simulink model "project_review_simulink"  (R2025b)
settings: Solver=ode4  StartTime=0.0  StopTime=5000  FixedStep=0.01  RelTol=1e-3
values from neighbouring files (symbols this model uses):
  a = 6900    [project_review.m]
  A_BN0 = eye(3)    [project_review.m]
  e = 0.01    [project_review.m]
  e_sun = deg2rad(23.45)    [project_review.m]
  inc = deg2rad(10)    [project_review.m]
  n = sqrt(mu_E / (a^3))    [project_review.m]
  n_sun = 2*pi / T_sun    (= 1.99102127766e-07)    [project_review.m]
  R_sun = 1.496e8    (= 149600000)    [project_review.m]
  sens_gyro_D_bias_inst = 0.3 / 3600    (= 8.33333333333e-05)    [project_review.m]
  sens_gyro_D_RW = sens_gyro_RRW / sqrt(3600)    [project_review.m]
  sens_gyro_D_wn = sens_gyro_D_ARW / sqrt(3600)    [project_review.m]
  sens_gyro_O = [1,      sens_gyro_eps_xy, sens_gyro_eps_xz ... (first row only)    [project_review.m]
  sens_gyro_run_run_bias = 4 / 3600    (= 0.00111111111111)    [project_review.m]
  sens_gyro_SFE = 500 * 1e-6    (= 0.0005)    [project_review.m]
  sens_gyro_SFN = 15 * 1e-6    (= 1.5e-05)    [project_review.m]
  sens_gyro_static_temp_bias = 9 / 3600    (= 0.0025)    [project_review.m]
  sens_gyro_theta_eps = [0,            -sens_gyro_theta_eps_z,  sens_gyro_theta_eps_y ... (first row only)    [project_review.m]
  sens_gyro_Ts = 1 / sens_gyro_update_rate    (= 0.01)    [project_review.m]
  TA0 = 0    [project_review.m]
undefined symbols (not defined in the file or in its folder): DiscIntNeverNeededParam
libraries: simulink_extras x3, perturbations x2, dynamics x1, kinematics x1, sensor_gyroscope x1
settings Model: Creator=nicol  LastModifiedBy=User

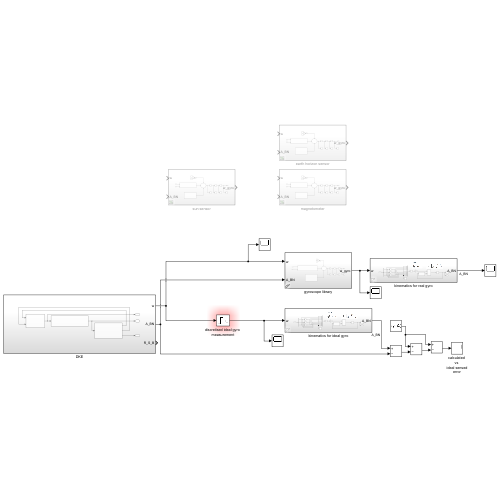
[thumbnail: Simulink's stored preview of the top-level diagram]
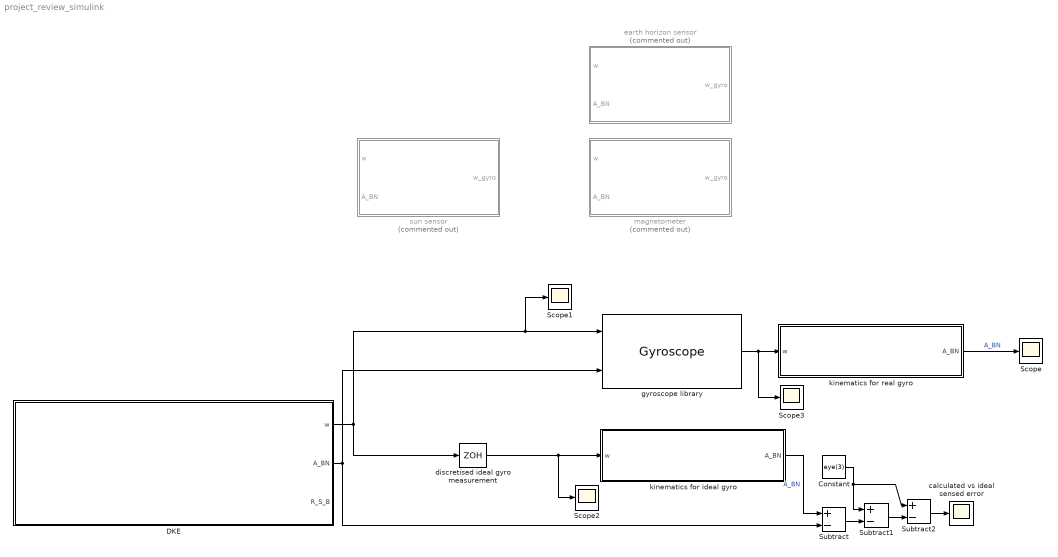
== system project_review_simulink ==
  Constant : Constant  Value=eye(3)
  DKE : Subsystem
  Scope{,1..3} (4 alike) : Scope
      Scope settings: ActiveDisplayYMinimum=-1.2499985302020951  ActiveDisplayYMaximum=1.2499998366891216  DataLoggingVariableName=ScopeData4
      Scope1 settings: ActiveDisplayYMinimum=-0.00077732778205415979  ActiveDisplayYMaximum=0.0013430338188456334  DataLoggingVariableName=ScopeData16
      Scope2 settings: ActiveDisplayYMinimum=-0.00029738297468781896  ActiveDisplayYMaximum=0.0013167850929970159  DataLoggingVariableName=ScopeData7
      Scope3 settings: ActiveDisplayYMinimum=-0.027987462414420936  ActiveDisplayYMaximum=0.080947574611551346  DataLoggingVariableName=ScopeData8
  Subtract : Sum  Inputs=+-
  Subtract1 : Sum  Inputs=+-
  Subtract2 : Sum  Inputs=+-
  calculated vs ideal sensed error : Scope
      settings: ActiveDisplayYMinimum=-2.47960605706532E-6  ActiveDisplayYMaximum=2.6662634592666823E-6  DataLoggingVariableName=ScopeData6
  discretised ideal gyro measurement : ZeroOrderHold  SampleTime=sens_gyro_Ts
  earth horizon sensor : Subsystem  Commented=on
  gyroscope library : sensor_gyroscope/Gyroscope  SystemSampleTime=-1  VariantActivationTime=update diagram  EmptyChoice=off  PassThrough=off  PassThroughVariantControl=(default)  EmptyChoiceVariantControl=(default)  AllowFlexibleInterface=on  Latency=0  AutoFrameSizeCalculation=off
  kinematics for ideal gyro : Subsystem  AncestorBlock=kinematics/kinematics
  kinematics for real gyro : Subsystem  AncestorBlock=kinematics/kinematics
  magnetometer : Subsystem  Commented=on
  sun sensor : Subsystem  Commented=on
  wires:
  DKE/1(w) -> discretised ideal gyro measurement/1, Scope1/1, gyroscope library/1
  gyroscope library/1 -> Scope3/1, kinematics for real gyro/1(w)
  discretised ideal gyro measurement/1 -> Scope2/1, kinematics for ideal gyro/1(w)
  kinematics for real gyro/1(A_BN) -> Scope/1  "A_BN"
  kinematics for ideal gyro/1(A_BN) -> Subtract/1  "A_BN"
  Subtract/1 -> Subtract1/2
  Constant/1 -> Subtract1/1, Subtract2/1
  Subtract1/1 -> Subtract2/2
  Subtract2/1 -> calculated vs ideal sensed error/1
  DKE/2(A_BN) -> Subtract/2, gyroscope library/2

== system project_review_simulink/DKE ==
  dynamics library : dynamics/dynamics  SystemSampleTime=-1  VariantActivationTime=update diagram  EmptyChoice=off  PassThrough=off  PassThroughVariantControl=(default)  EmptyChoiceVariantControl=(default)  AllowFlexibleInterface=on  Latency=0  AutoFrameSizeCalculation=off
  environment : Subsystem
  kinematics library : kinematics/kinematics  SystemSampleTime=-1  VariantActivationTime=update diagram  EmptyChoice=off  PassThrough=off  PassThroughVariantControl=(default)  EmptyChoiceVariantControl=(default)  AllowFlexibleInterface=on  Latency=0  AutoFrameSizeCalculation=off
  w : Outport
  A_BN : Outport  Port=2
  R_S_B : Outport  Port=3
  wires:
  dynamics library/1 -> w/1, kinematics library/1
  kinematics library/1 -> A_BN/1, environment/1(A_BN)
  environment/1(gravity gradient torque) -> dynamics library/1
  environment/2(magnetic torque) -> dynamics library/2
  environment/3(R_S_B) -> R_S_B/1  "position of sun  in body frame"

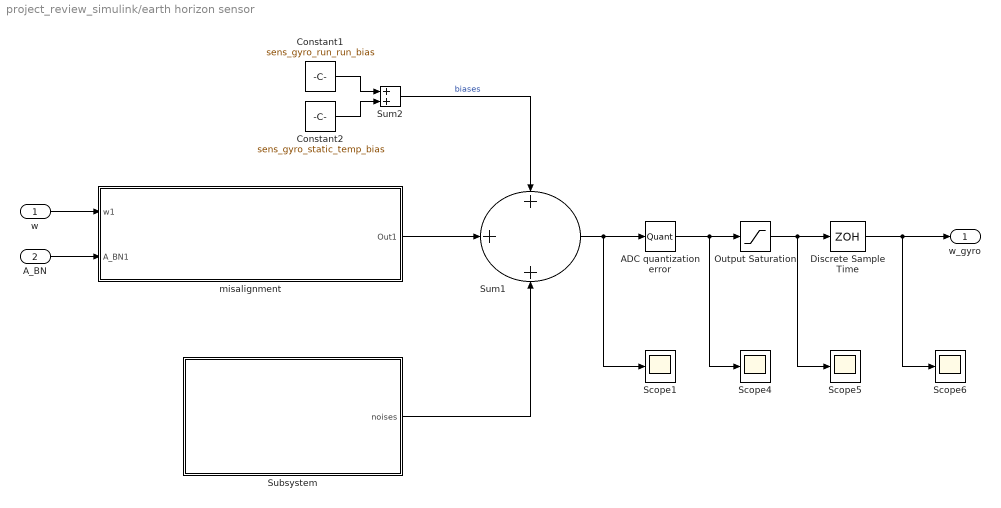
== system project_review_simulink/earth horizon sensor ==
  w : Inport
  A_BN : Inport  Port=2
  ADC quantization error : Quantizer  QuantizationInterval=sens_gyro_LSB
  Constant1 : Constant  Value=sens_gyro_run_run_bias
  Constant2 : Constant  Value=sens_gyro_static_temp_bias
  Discrete Sample Time : ZeroOrderHold  SampleTime=sens_gyro_Ts
  Output Saturation : Saturate  UpperLimit=20  LowerLimit=-20
  Scope{1,4..6} (4 alike) : Scope
      Scope1 settings: ActiveDisplayYMinimum=-0.032120647567430112  ActiveDisplayYMaximum=0.096644162809020939  DataLoggingVariableName=ScopeData9
      Scope4 settings: ActiveDisplayYMinimum=-1  ActiveDisplayYMaximum=1  DataLoggingVariableName=ScopeData10
      Scope5 settings: ActiveDisplayYMinimum=-1  ActiveDisplayYMaximum=1  DataLoggingVariableName=ScopeData11
      Scope6 settings: ActiveDisplayYMinimum=-0.032120647471039  ActiveDisplayYMaximum=0.096644162883216228  DataLoggingVariableName=ScopeData12
  Subsystem : Subsystem
  Sum1 : Sum  Inputs=+++
  Sum2 : Sum
  misalignment : Subsystem
  w_gyro : Outport
  wires:
  Constant1/1 -> Sum2/1
  A_BN/1 -> misalignment/2(A_BN1)
  Subsystem/1(noises) -> Sum1/3
  w/1 -> misalignment/1(w1)
  Output Saturation/1 -> Scope5/1, Discrete Sample Time/1
  Sum2/1 -> Sum1/1  "biases"
  ADC quantization error/1 -> Scope4/1, Output Saturation/1
  Sum1/1 -> Scope1/1, ADC quantization error/1
  Discrete Sample Time/1 -> w_gyro/1, Scope6/1
  Constant2/1 -> Sum2/2
  misalignment/1(Out1) -> Sum1/2

== system project_review_simulink/kinematics for ideal gyro ==
  w : Inport
  Constant2 : Constant  Value=0
  Demux : Demux  Outputs=3
  Gain{8..11} (4 alike) : Gain  Gain=-1
  Integrator5 : Integrator  InitialCondition=A_BN0
  Product5 : Product  Multiplication=Matrix(*)
  Reshape2 : Reshape  OutputDimensionality=Customize  OutputDimensions=[3,3]
  Scope1 : Scope
      settings: ActiveDisplayYMinimum=-1.2499999998899596  ActiveDisplayYMaximum=1.2499999999877733
  Vector Concatenate2 : Concatenate  NumInputs=9
  orthonormalisation : Subsystem
  A_BN : Outport
  wires:
  orthonormalisation/1(" A_BN") -> Product5/2
  w/1 -> Demux/1
  Gain9/1 -> Vector Concatenate2/8  "-wx"
  Constant2/1 -> Vector Concatenate2/9, Vector Concatenate2/5, Vector Concatenate2/1  "0"
  Demux/3 -> Gain11/1, Vector Concatenate2/2  "wz"
  Vector Concatenate2/1 -> Reshape2/1
  Demux/2 -> Gain10/1, Vector Concatenate2/7  "wy"
  Gain10/1 -> Vector Concatenate2/3  "-wy"
  Reshape2/1 -> Gain8/1
  Demux/1 -> Gain9/1, Vector Concatenate2/6  "wx"
  Gain8/1 -> Product5/1
  Integrator5/1 -> orthonormalisation/1(A_BN), Scope1/1, A_BN/1  "A_BN"
  Gain11/1 -> Vector Concatenate2/4  "-wz"
  Product5/1 -> Integrator5/1  "dA_BN(t)/dt"

== system project_review_simulink/kinematics for real gyro ==
  w : Inport
  Constant2 : Constant  Value=0
  Demux : Demux  Outputs=3
  Gain{8..11} (4 alike) : Gain  Gain=-1
  Integrator5 : Integrator  InitialCondition=A_BN0
  Product5 : Product  Multiplication=Matrix(*)
  Reshape2 : Reshape  OutputDimensionality=Customize  OutputDimensions=[3,3]
  Scope1 : Scope
      settings: ActiveDisplayYMinimum=-1.2499999998899596  ActiveDisplayYMaximum=1.2499999999877733
  Vector Concatenate2 : Concatenate  NumInputs=9
  orthonormalisation : Subsystem
  A_BN : Outport
  wires:
  Product5/1 -> Integrator5/1  "dA_BN(t)/dt"
  Gain11/1 -> Vector Concatenate2/4  "-wz"
  Integrator5/1 -> A_BN/1, Scope1/1, orthonormalisation/1(A_BN)  "A_BN"
  Gain8/1 -> Product5/1
  Demux/1 -> Vector Concatenate2/6, Gain9/1  "wx"
  Reshape2/1 -> Gain8/1
  Gain10/1 -> Vector Concatenate2/3  "-wy"
  Demux/2 -> Vector Concatenate2/7, Gain10/1  "wy"
  Vector Concatenate2/1 -> Reshape2/1
  Demux/3 -> Vector Concatenate2/2, Gain11/1  "wz"
  Constant2/1 -> Vector Concatenate2/1, Vector Concatenate2/5, Vector Concatenate2/9  "0"
  Gain9/1 -> Vector Concatenate2/8  "-wx"
  w/1 -> Demux/1
  orthonormalisation/1(" A_BN") -> Product5/2

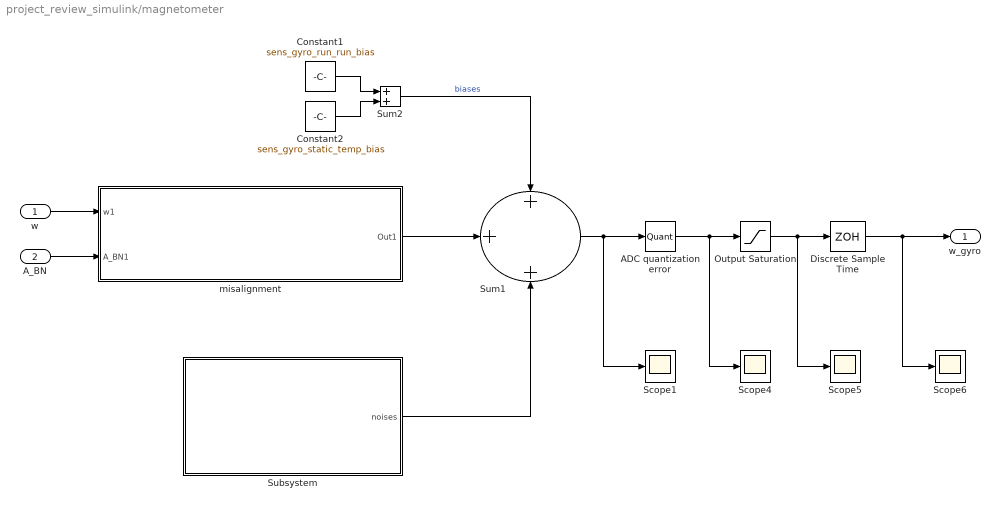
== system project_review_simulink/magnetometer ==
  w : Inport
  A_BN : Inport  Port=2
  ADC quantization error : Quantizer  QuantizationInterval=sens_gyro_LSB
  Constant1 : Constant  Value=sens_gyro_run_run_bias
  Constant2 : Constant  Value=sens_gyro_static_temp_bias
  Discrete Sample Time : ZeroOrderHold  SampleTime=sens_gyro_Ts
  Output Saturation : Saturate  UpperLimit=20  LowerLimit=-20
  Scope{1,4..6} (4 alike) : Scope
      Scope1 settings: ActiveDisplayYMinimum=-0.032120647567430112  ActiveDisplayYMaximum=0.096644162809020939  DataLoggingVariableName=ScopeData9
      Scope4 settings: ActiveDisplayYMinimum=-1  ActiveDisplayYMaximum=1  DataLoggingVariableName=ScopeData10
      Scope5 settings: ActiveDisplayYMinimum=-1  ActiveDisplayYMaximum=1  DataLoggingVariableName=ScopeData11
      Scope6 settings: ActiveDisplayYMinimum=-0.032120647471039  ActiveDisplayYMaximum=0.096644162883216228  DataLoggingVariableName=ScopeData12
  Subsystem : Subsystem
  Sum1 : Sum  Inputs=+++
  Sum2 : Sum
  misalignment : Subsystem
  w_gyro : Outport
  wires:
  Constant1/1 -> Sum2/1
  A_BN/1 -> misalignment/2(A_BN1)
  Subsystem/1(noises) -> Sum1/3
  w/1 -> misalignment/1(w1)
  Output Saturation/1 -> Scope5/1, Discrete Sample Time/1
  Sum2/1 -> Sum1/1  "biases"
  ADC quantization error/1 -> Scope4/1, Output Saturation/1
  Sum1/1 -> Scope1/1, ADC quantization error/1
  Discrete Sample Time/1 -> w_gyro/1, Scope6/1
  Constant2/1 -> Sum2/2
  misalignment/1(Out1) -> Sum1/2

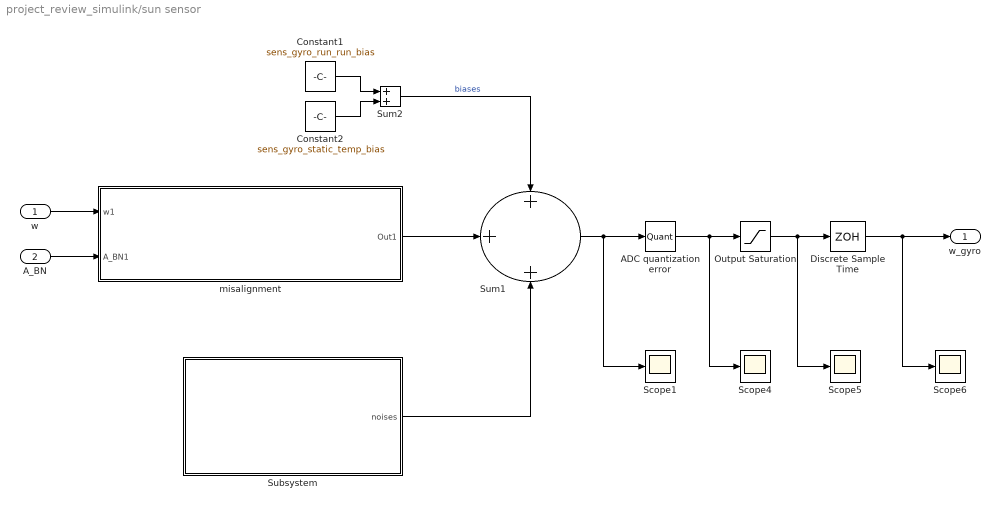
== system project_review_simulink/sun sensor ==
  w : Inport
  A_BN : Inport  Port=2
  ADC quantization error : Quantizer  QuantizationInterval=sens_gyro_LSB
  Constant1 : Constant  Value=sens_gyro_run_run_bias
  Constant2 : Constant  Value=sens_gyro_static_temp_bias
  Discrete Sample Time : ZeroOrderHold  SampleTime=sens_gyro_Ts
  Output Saturation : Saturate  UpperLimit=20  LowerLimit=-20
  Scope{1,4..6} (4 alike) : Scope
      Scope1 settings: ActiveDisplayYMinimum=-0.032120647567430112  ActiveDisplayYMaximum=0.096644162809020939  DataLoggingVariableName=ScopeData9
      Scope4 settings: ActiveDisplayYMinimum=-1  ActiveDisplayYMaximum=1  DataLoggingVariableName=ScopeData10
      Scope5 settings: ActiveDisplayYMinimum=-1  ActiveDisplayYMaximum=1  DataLoggingVariableName=ScopeData11
      Scope6 settings: ActiveDisplayYMinimum=-0.032120647471039  ActiveDisplayYMaximum=0.096644162883216228  DataLoggingVariableName=ScopeData12
  Subsystem : Subsystem
  Sum1 : Sum  Inputs=+++
  Sum2 : Sum
  misalignment : Subsystem
  w_gyro : Outport
  wires:
  misalignment/1(Out1) -> Sum1/2
  Constant2/1 -> Sum2/2
  Discrete Sample Time/1 -> Scope6/1, w_gyro/1
  Sum1/1 -> ADC quantization error/1, Scope1/1
  ADC quantization error/1 -> Output Saturation/1, Scope4/1
  Sum2/1 -> Sum1/1  "biases"
  Output Saturation/1 -> Discrete Sample Time/1, Scope5/1
  w/1 -> misalignment/1(w1)
  Subsystem/1(noises) -> Sum1/3
  A_BN/1 -> misalignment/2(A_BN1)
  Constant1/1 -> Sum2/1

== system project_review_simulink/DKE/environment ==
  A_BN : Inport
  Matrix Multiply : Product  Multiplication=Matrix(*)
  compute sun position in inertial frame : Subsystem
  magnetic torque library : perturbations/magnetic torque  SystemSampleTime=-1  VariantActivationTime=update diagram  EmptyChoice=off  PassThrough=off  PassThroughVariantControl=(default)  EmptyChoiceVariantControl=(default)  AllowFlexibleInterface=on  Latency=0  AutoFrameSizeCalculation=off
  non-circular gravity gradient library : perturbations/non-circular gravity gradient  SystemSampleTime=-1  VariantActivationTime=update diagram  EmptyChoice=off  PassThrough=off  PassThroughVariantControl=(default)  EmptyChoiceVariantControl=(default)  AllowFlexibleInterface=on  Latency=0  AutoFrameSizeCalculation=off
      settings: PortSchema="{\"entries\":[{\"content\":{\"sides\":[{\"content\":{\"connectorIds\":[\"Out1\"]},\"type\":\"ConnectorPlacement.EquallySpacedRectSide\",\"uuid\":\"2a67419a-68c9-4369-a698-e6ac26417455\"},{\"content\":{\"connectorIds\":[\"In1\",\"In2\"],\"side\":\"RIGHT\"},\"type\":\"ConnectorPlacement.EquallySpacedRectSide\",\"uuid\":\"5f3f4c4a-6b79-4b92-8f4c-19ffa36753b2\"},{\"content\":{\"side\":\"TOP\"},\"type\":\"ConnectorPlacement.EquallySpacedRectSide\",\"uuid\":\"22c946b7-ea77-4444-a63c-d5b3d585f671\"}]},\"type\":\"ConnectorPlacement.EquallySpacedConnector\",\"uuid\":\"037c4a72-b28b-418e-a921-9da68dc0cd93\"}],\"packageUris\":[\"http://schema.mathworks.com/mf0/Connector/R2020b\"],\"version\":\"1.0\"}"
  position and attitude : Subsystem
  gravity gradient torque : Outport
  magnetic torque : Outport  Port=2
  R_S_B : Outport  Port=3
  wires:
  A_BN/1 -> position and attitude/1(A_BN), Matrix Multiply/1, magnetic torque library/1
  non-circular gravity gradient library/1 -> gravity gradient torque/1  "GG torque"
  magnetic torque library/1 -> magnetic torque/1  "M torque"
  position and attitude/1(r_N) -> magnetic torque library/2, non-circular gravity gradient library/2
  position and attitude/3(A_BL) -> non-circular gravity gradient library/1
  position and attitude/2(r) -> magnetic torque library/3
  compute sun position in inertial frame/1(R_S_N) -> Matrix Multiply/2
  Matrix Multiply/1 -> R_S_B/1

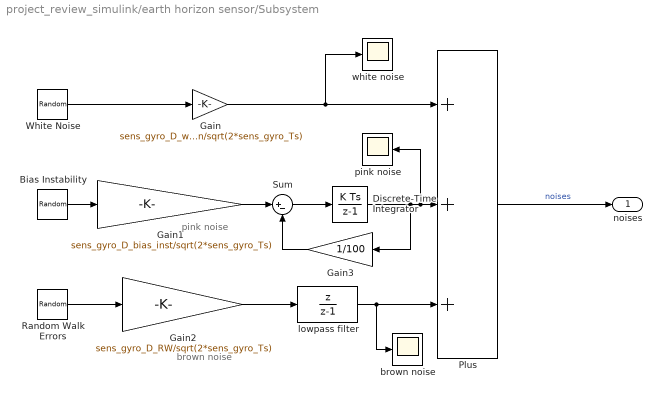
== system project_review_simulink/earth horizon sensor/Subsystem ==
  note: brown noise
  note: pink noise
  " White Noise" : RandomNumber  SampleTime=0.1
  Bias Instability : RandomNumber  SampleTime=0.1
  Discrete-Time Integrator : DiscreteIntegrator  ICPrevOutput=DiscIntNeverNeededParam  ICPrevScaledInput=DiscIntNeverNeededParam
  Gain : Gain  Gain=sens_gyro_D_wn/sqrt(2*sens_gyro_Ts)
  Gain1 : Gain  Gain=sens_gyro_D_bias_inst/sqrt(2*sens_gyro_Ts)
  Gain2 : Gain  Gain=sens_gyro_D_RW/sqrt(2*sens_gyro_Ts)
  Gain3 : Gain  Gain=1/100
  Plus : Sum  Inputs=+++
  Random Walk Errors : RandomNumber  SampleTime=0.1
  Sum : Sum  Inputs=|+-
  brown noise : Scope
      settings: ActiveDisplayYMinimum=-0.025691906984189852  ActiveDisplayYMaximum=0.0025755592198982418  DataLoggingVariableName=ScopeData13
  lowpass filter : DiscreteTransferFcn  Numerator=[1 0]  Denominator=[1 -1]
  pink noise : Scope
      settings: ActiveDisplayYMinimum=-0.013777619312277414  ActiveDisplayYMaximum=0.014220901201123974  DataLoggingVariableName=ScopeData14
  white noise : Scope
      settings: ActiveDisplayYMinimum=-0.0017013348354620785  ActiveDisplayYMaximum=0.001720930099973718  DataLoggingVariableName=ScopeData15
  noises : Outport
  wires:
  Gain3/1 -> Sum/2
  " White Noise"/1 -> Gain/1
  Gain/1 -> white noise/1, Plus/1
  Bias Instability/1 -> Gain1/1
  Discrete-Time Integrator/1 -> pink noise/1, Plus/2, Gain3/1
  Plus/1 -> noises/1  "noises"
  Gain2/1 -> lowpass filter/1
  Gain1/1 -> Sum/1
  Sum/1 -> Discrete-Time Integrator/1
  lowpass filter/1 -> Plus/3, brown noise/1
  Random Walk Errors/1 -> Gain2/1

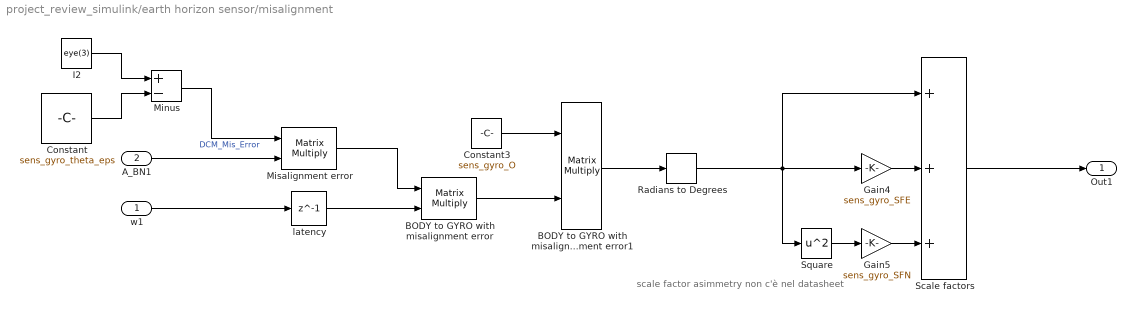
== system project_review_simulink/earth horizon sensor/misalignment ==
  note: scale factor asimmetry non c'è nel datasheet
  w1 : Inport
  A_BN1 : Inport  Port=2
  BODY to GYRO with misalignment error : Product  Multiplication=Matrix(*)
  BODY to GYRO with misalignment error1 : Product  Multiplication=Matrix(*)
  Constant : Constant  Value=sens_gyro_theta_eps
  Constant3 : Constant  Value=sens_gyro_O
  Gain4 : Gain  Gain=sens_gyro_SFE
  Gain5 : Gain  Gain=sens_gyro_SFN
  I2 : Constant  Value=eye(3)
  Minus : Sum  Inputs=+-
  Misalignment error : Product  Multiplication=Matrix(*)
  Radians to Degrees : simulink_extras/Transformations/Radians to Degrees
  Scale factors : Sum  Inputs=+++
  Square : Math  Operator=square
  latency : Delay  DelayLength=1
  Out1 : Outport
  wires:
  Misalignment error/1 -> BODY to GYRO with misalignment error/1
  latency/1 -> BODY to GYRO with misalignment error/2
  BODY to GYRO with misalignment error1/1 -> Radians to Degrees/1
  A_BN1/1 -> Misalignment error/2
  Constant3/1 -> BODY to GYRO with misalignment error1/1
  Square/1 -> Gain5/1
  Gain4/1 -> Scale factors/2
  Radians to Degrees/1 -> Scale factors/1, Gain4/1, Square/1
  I2/1 -> Minus/1
  Minus/1 -> Misalignment error/1  "DCM_Mis_Error"
  BODY to GYRO with misalignment error/1 -> BODY to GYRO with misalignment error1/2
  w1/1 -> latency/1
  Scale factors/1 -> Out1/1
  Gain5/1 -> Scale factors/3
  Constant/1 -> Minus/2

== system project_review_simulink/kinematics for ideal gyro/orthonormalisation ==
  A_BN : Inport
  Gain : Gain  Gain=3/2
  Gain1 : Gain  Gain=1/2
  Matrix Multiply1 : Product  Inputs=3  Multiplication=Matrix(*)
  Subtract : Sum  Inputs=+-
  Transpose1 : Math  Operator=transpose
  " A_BN" : Outport
  wires:
  A_BN/1 -> Matrix Multiply1/3, Transpose1/1, Gain/1, Matrix Multiply1/1
  Subtract/1 -> " A_BN"/1
  Gain1/1 -> Subtract/2
  Matrix Multiply1/1 -> Gain1/1
  Transpose1/1 -> Matrix Multiply1/2
  Gain/1 -> Subtract/1

== system project_review_simulink/kinematics for real gyro/orthonormalisation ==
  A_BN : Inport
  Gain : Gain  Gain=3/2
  Gain1 : Gain  Gain=1/2
  Matrix Multiply1 : Product  Inputs=3  Multiplication=Matrix(*)
  Subtract : Sum  Inputs=+-
  Transpose1 : Math  Operator=transpose
  " A_BN" : Outport
  wires:
  Gain/1 -> Subtract/1
  Transpose1/1 -> Matrix Multiply1/2
  Matrix Multiply1/1 -> Gain1/1
  Gain1/1 -> Subtract/2
  Subtract/1 -> " A_BN"/1
  A_BN/1 -> Matrix Multiply1/1, Gain/1, Transpose1/1, Matrix Multiply1/3

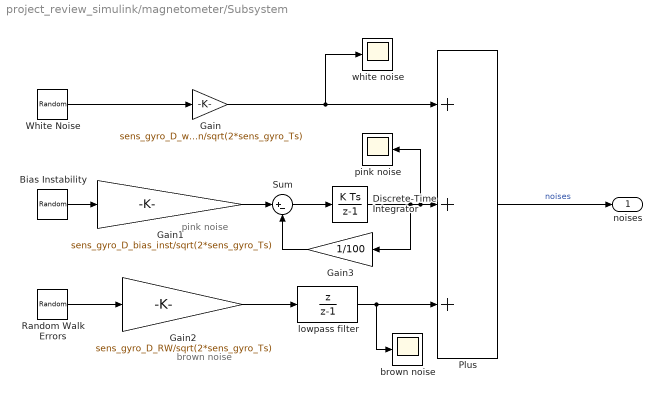
== system project_review_simulink/magnetometer/Subsystem ==
  note: brown noise
  note: pink noise
  " White Noise" : RandomNumber  SampleTime=0.1
  Bias Instability : RandomNumber  SampleTime=0.1
  Discrete-Time Integrator : DiscreteIntegrator  ICPrevOutput=DiscIntNeverNeededParam  ICPrevScaledInput=DiscIntNeverNeededParam
  Gain : Gain  Gain=sens_gyro_D_wn/sqrt(2*sens_gyro_Ts)
  Gain1 : Gain  Gain=sens_gyro_D_bias_inst/sqrt(2*sens_gyro_Ts)
  Gain2 : Gain  Gain=sens_gyro_D_RW/sqrt(2*sens_gyro_Ts)
  Gain3 : Gain  Gain=1/100
  Plus : Sum  Inputs=+++
  Random Walk Errors : RandomNumber  SampleTime=0.1
  Sum : Sum  Inputs=|+-
  brown noise : Scope
      settings: ActiveDisplayYMinimum=-0.025691906984189852  ActiveDisplayYMaximum=0.0025755592198982418  DataLoggingVariableName=ScopeData13
  lowpass filter : DiscreteTransferFcn  Numerator=[1 0]  Denominator=[1 -1]
  pink noise : Scope
      settings: ActiveDisplayYMinimum=-0.013777619312277414  ActiveDisplayYMaximum=0.014220901201123974  DataLoggingVariableName=ScopeData14
  white noise : Scope
      settings: ActiveDisplayYMinimum=-0.0017013348354620785  ActiveDisplayYMaximum=0.001720930099973718  DataLoggingVariableName=ScopeData15
  noises : Outport
  wires:
  Gain3/1 -> Sum/2
  " White Noise"/1 -> Gain/1
  Gain/1 -> white noise/1, Plus/1
  Bias Instability/1 -> Gain1/1
  Discrete-Time Integrator/1 -> pink noise/1, Plus/2, Gain3/1
  Plus/1 -> noises/1  "noises"
  Gain2/1 -> lowpass filter/1
  Gain1/1 -> Sum/1
  Sum/1 -> Discrete-Time Integrator/1
  lowpass filter/1 -> Plus/3, brown noise/1
  Random Walk Errors/1 -> Gain2/1

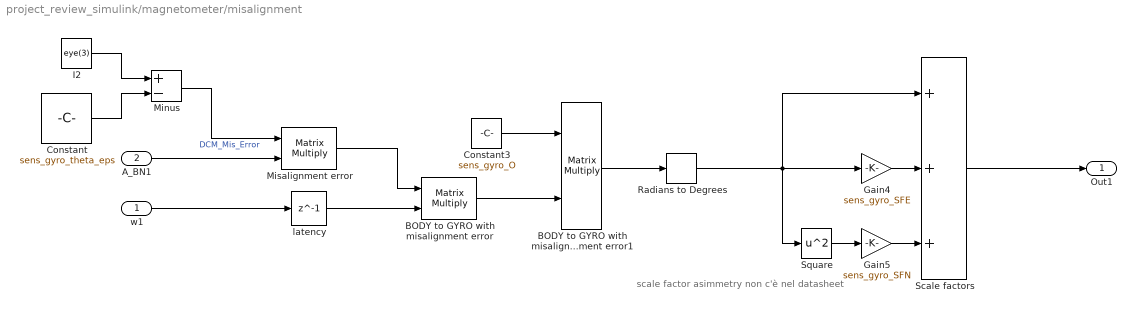
== system project_review_simulink/magnetometer/misalignment ==
  note: scale factor asimmetry non c'è nel datasheet
  w1 : Inport
  A_BN1 : Inport  Port=2
  BODY to GYRO with misalignment error : Product  Multiplication=Matrix(*)
  BODY to GYRO with misalignment error1 : Product  Multiplication=Matrix(*)
  Constant : Constant  Value=sens_gyro_theta_eps
  Constant3 : Constant  Value=sens_gyro_O
  Gain4 : Gain  Gain=sens_gyro_SFE
  Gain5 : Gain  Gain=sens_gyro_SFN
  I2 : Constant  Value=eye(3)
  Minus : Sum  Inputs=+-
  Misalignment error : Product  Multiplication=Matrix(*)
  Radians to Degrees : simulink_extras/Transformations/Radians to Degrees
  Scale factors : Sum  Inputs=+++
  Square : Math  Operator=square
  latency : Delay  DelayLength=1
  Out1 : Outport
  wires:
  Misalignment error/1 -> BODY to GYRO with misalignment error/1
  latency/1 -> BODY to GYRO with misalignment error/2
  BODY to GYRO with misalignment error1/1 -> Radians to Degrees/1
  A_BN1/1 -> Misalignment error/2
  Constant3/1 -> BODY to GYRO with misalignment error1/1
  Square/1 -> Gain5/1
  Gain4/1 -> Scale factors/2
  Radians to Degrees/1 -> Scale factors/1, Gain4/1, Square/1
  I2/1 -> Minus/1
  Minus/1 -> Misalignment error/1  "DCM_Mis_Error"
  BODY to GYRO with misalignment error/1 -> BODY to GYRO with misalignment error1/2
  w1/1 -> latency/1
  Scale factors/1 -> Out1/1
  Gain5/1 -> Scale factors/3
  Constant/1 -> Minus/2

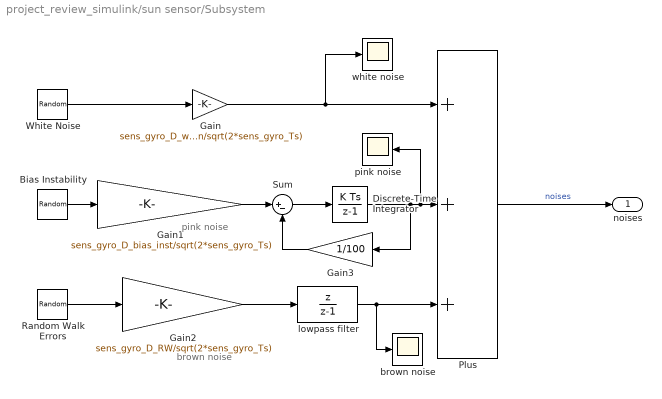
== system project_review_simulink/sun sensor/Subsystem ==
  note: pink noise
  note: brown noise
  " White Noise" : RandomNumber  SampleTime=0.1
  Bias Instability : RandomNumber  SampleTime=0.1
  Discrete-Time Integrator : DiscreteIntegrator  ICPrevOutput=DiscIntNeverNeededParam  ICPrevScaledInput=DiscIntNeverNeededParam
  Gain : Gain  Gain=sens_gyro_D_wn/sqrt(2*sens_gyro_Ts)
  Gain1 : Gain  Gain=sens_gyro_D_bias_inst/sqrt(2*sens_gyro_Ts)
  Gain2 : Gain  Gain=sens_gyro_D_RW/sqrt(2*sens_gyro_Ts)
  Gain3 : Gain  Gain=1/100
  Plus : Sum  Inputs=+++
  Random Walk Errors : RandomNumber  SampleTime=0.1
  Sum : Sum  Inputs=|+-
  brown noise : Scope
      settings: ActiveDisplayYMinimum=-0.025691906984189852  ActiveDisplayYMaximum=0.0025755592198982418  DataLoggingVariableName=ScopeData13
  lowpass filter : DiscreteTransferFcn  Numerator=[1 0]  Denominator=[1 -1]
  pink noise : Scope
      settings: ActiveDisplayYMinimum=-0.013777619312277414  ActiveDisplayYMaximum=0.014220901201123974  DataLoggingVariableName=ScopeData14
  white noise : Scope
      settings: ActiveDisplayYMinimum=-0.0017013348354620785  ActiveDisplayYMaximum=0.001720930099973718  DataLoggingVariableName=ScopeData15
  noises : Outport
  wires:
  Random Walk Errors/1 -> Gain2/1
  lowpass filter/1 -> brown noise/1, Plus/3
  Sum/1 -> Discrete-Time Integrator/1
  Gain1/1 -> Sum/1
  Gain2/1 -> lowpass filter/1
  Plus/1 -> noises/1  "noises"
  Discrete-Time Integrator/1 -> Gain3/1, Plus/2, pink noise/1
  Bias Instability/1 -> Gain1/1
  Gain/1 -> Plus/1, white noise/1
  " White Noise"/1 -> Gain/1
  Gain3/1 -> Sum/2

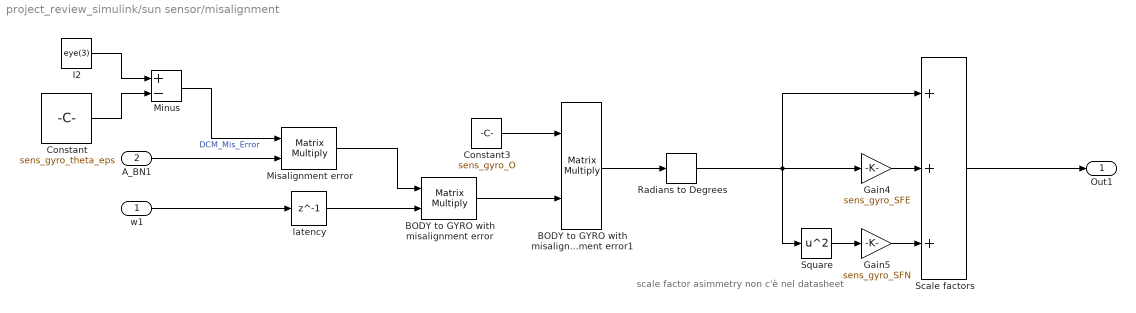
== system project_review_simulink/sun sensor/misalignment ==
  note: scale factor asimmetry non c'è nel datasheet
  w1 : Inport
  A_BN1 : Inport  Port=2
  BODY to GYRO with misalignment error : Product  Multiplication=Matrix(*)
  BODY to GYRO with misalignment error1 : Product  Multiplication=Matrix(*)
  Constant : Constant  Value=sens_gyro_theta_eps
  Constant3 : Constant  Value=sens_gyro_O
  Gain4 : Gain  Gain=sens_gyro_SFE
  Gain5 : Gain  Gain=sens_gyro_SFN
  I2 : Constant  Value=eye(3)
  Minus : Sum  Inputs=+-
  Misalignment error : Product  Multiplication=Matrix(*)
  Radians to Degrees : simulink_extras/Transformations/Radians to Degrees
  Scale factors : Sum  Inputs=+++
  Square : Math  Operator=square
  latency : Delay  DelayLength=1
  Out1 : Outport
  wires:
  Constant/1 -> Minus/2
  Gain5/1 -> Scale factors/3
  Scale factors/1 -> Out1/1
  w1/1 -> latency/1
  BODY to GYRO with misalignment error/1 -> BODY to GYRO with misalignment error1/2
  Minus/1 -> Misalignment error/1  "DCM_Mis_Error"
  I2/1 -> Minus/1
  Radians to Degrees/1 -> Square/1, Gain4/1, Scale factors/1
  Gain4/1 -> Scale factors/2
  Square/1 -> Gain5/1
  Constant3/1 -> BODY to GYRO with misalignment error1/1
  A_BN1/1 -> Misalignment error/2
  BODY to GYRO with misalignment error1/1 -> Radians to Degrees/1
  latency/1 -> BODY to GYRO with misalignment error/2
  Misalignment error/1 -> BODY to GYRO with misalignment error/1

== system project_review_simulink/DKE/environment/compute sun position in inertial frame ==
  Clock : Clock
  Constant : Constant  Value=n_sun
  Constant1 : Constant  Value=e_sun
  Cos : Trigonometry  Operator=cos
  Cos1 : Trigonometry  Operator=cos
  Gain : Gain  Gain=R_sun
  Mux : Mux  Inputs=3
  Product : Product
  Product1 : Product
  Product2 : Product
  Scope2 : Scope
      settings: ActiveDisplayYMinimum=-1.8699999999999996E+7  ActiveDisplayYMaximum=1.683E+8  DataLoggingVariableName=ScopeData17
  Sin : Trigonometry
  Sin2 : Trigonometry
  To Workspace2 : ToWorkspace  VariableName=S_N  SaveFormat=Timeseries  SampleTime=-1
  R_S_N : Outport
  wires:
  Constant/1 -> Product/2
  Sin/1 -> Product1/1, Product2/1
  Product1/1 -> Mux/2
  Clock/1 -> Product/1
  Gain/1 -> R_S_N/1, To Workspace2/1, Scope2/1
  Mux/1 -> Gain/1
  Sin2/1 -> Product2/2
  Cos1/1 -> Mux/1
  Cos/1 -> Product1/2
  Product2/1 -> Mux/3
  Product/1 -> Cos1/1, Sin/1
  Constant1/1 -> Sin2/1, Cos/1

== system project_review_simulink/DKE/environment/position and attitude ==
  A_BN : Inport
  Constant : Constant  Value=inc
  compute position : Subsystem
  non-circular reference attitude : Subsystem
  r_N : Outport
  r : Outport  Port=2
  A_BL : Outport  Port=3
  wires:
  compute position/3(TA) -> non-circular reference attitude/1(TA)
  compute position/1(r_N) -> r_N/1
  Constant/1 -> non-circular reference attitude/2(i)
  compute position/2(r) -> r/1
  A_BN/1 -> non-circular reference attitude/3(A_BN)
  non-circular reference attitude/1(A_BL) -> A_BL/1

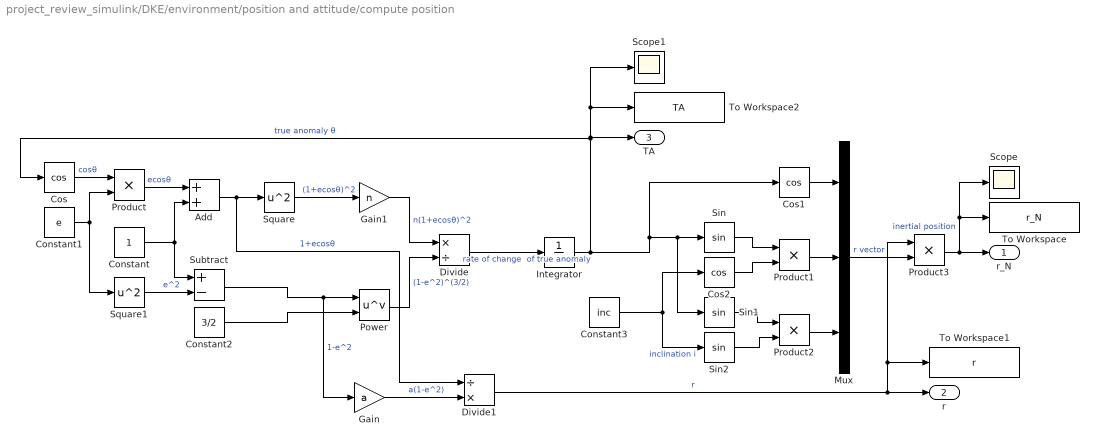
== system project_review_simulink/DKE/environment/position and attitude/compute position ==
  Add : Sum
  Constant : Constant
  Constant1 : Constant  Value=e
  Constant2 : Constant  Value=3/2
  Constant3 : Constant  Value=inc
  Cos : Trigonometry  Operator=cos
  Cos1 : Trigonometry  Operator=cos
  Cos2 : Trigonometry  Operator=cos
  Divide : Product  Inputs=*/
  Divide1 : Product  Inputs=/*
  Gain : Gain  Gain=a
  Gain1 : Gain  Gain=n
  Integrator : Integrator  InitialCondition=TA0
  Mux : Mux  Inputs=3
  Power : Math  Operator=pow
  Product{,1..3} (4 alike) : Product
  Scope : Scope
      settings: ActiveDisplayYMinimum=-1  ActiveDisplayYMaximum=1  DataLoggingVariableName=ScopeData3
  Scope1 : Scope
      settings: ActiveDisplayYMinimum=-1  ActiveDisplayYMaximum=1  DataLoggingVariableName=ScopeData5
  Sin : Trigonometry
  Sin1 : Trigonometry
  Sin2 : Trigonometry
  Square : Math  Operator=square
  Square1 : Math  Operator=square
  Subtract : Sum  Inputs=+-
  To Workspace : ToWorkspace  VariableName=r_N  SaveFormat=Timeseries  SampleTime=-1
  To Workspace1 : ToWorkspace  VariableName=r  SaveFormat=Timeseries  SampleTime=-1
  To Workspace2 : ToWorkspace  VariableName=TA  SaveFormat=Timeseries  SampleTime=-1
  r_N : Outport
  r : Outport  Port=2
  TA : Outport  Port=3
  wires:
  Integrator/1 -> Sin1/1, Sin/1, Cos1/1, TA/1, Scope1/1, To Workspace2/1, Cos/1  "true anomaly θ"
  Add/1 -> Divide1/1, Square/1  "1+ecosθ"
  Square/1 -> Gain1/1  "(1+ecosθ)^2"
  Gain1/1 -> Divide/1  "n(1+ecosθ)^2"
  Sin1/1 -> Product2/1
  Constant/1 -> Subtract/1, Add/2
  Subtract/1 -> Gain/1, Power/1  "1-e^2"
  Product3/1 -> r_N/1, To Workspace/1, Scope/1  "inertial position"
  Constant3/1 -> Cos2/1, Sin2/1  "inclination i"
  Gain/1 -> Divide1/2  "a(1-e^2)"
  Constant2/1 -> Power/2
  Sin2/1 -> Product2/2
  Cos/1 -> Product/1  "cosθ"
  Constant1/1 -> Square1/1, Product/2
  Product/1 -> Add/1  "ecosθ"
  Product2/1 -> Mux/3
  Square1/1 -> Subtract/2  "e^2"
  Divide1/1 -> Product3/1, To Workspace1/1, r/1  "r"
  Cos1/1 -> Mux/1
  Mux/1 -> Product3/2  "r vector"
  Power/1 -> Divide/2  "(1-e^2)^(3/2)"
  Product1/1 -> Mux/2
  Divide/1 -> Integrator/1  "rate of change  of true anomaly"
  Sin/1 -> Product1/1
  Cos2/1 -> Product1/2

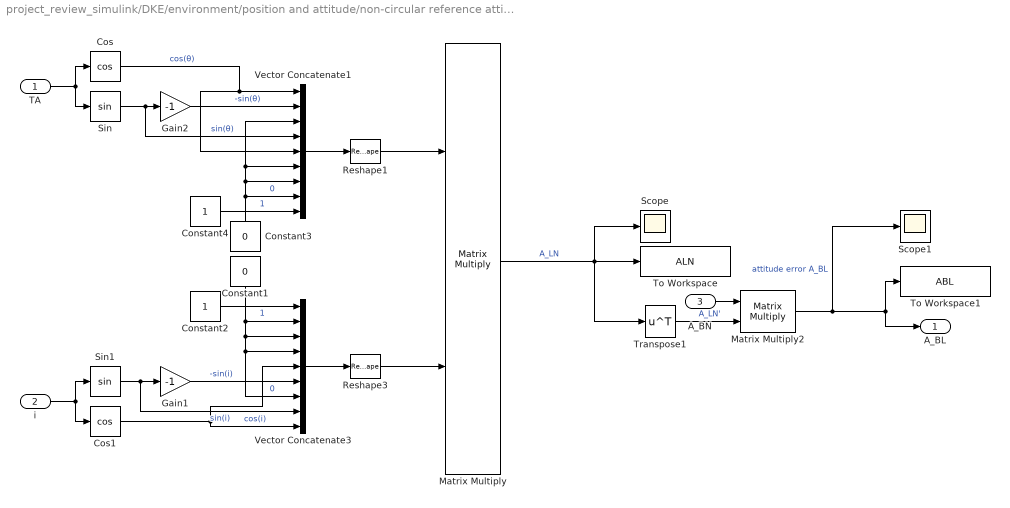
== system project_review_simulink/DKE/environment/position and attitude/non-circular reference attitude ==
  TA : Inport
  i : Inport  Port=2
  A_BN : Inport  Port=3
  Constant1 : Constant  Value=0
  Constant2 : Constant
  Constant3 : Constant  Value=0
  Constant4 : Constant
  Cos : Trigonometry  Operator=cos
  Cos1 : Trigonometry  Operator=cos
  Gain1 : Gain  Gain=-1
  Gain2 : Gain  Gain=-1
  Matrix Multiply : Product  Multiplication=Matrix(*)
  Matrix Multiply2 : Product  Multiplication=Matrix(*)
  Reshape1 : Reshape  OutputDimensionality=Customize  OutputDimensions=[3,3]
  Reshape3 : Reshape  OutputDimensionality=Customize  OutputDimensions=[3,3]
  Scope : Scope
      settings: ActiveDisplayYMinimum=-1.2383013929227509  ActiveDisplayYMaximum=1.2487001547691945  DataLoggingVariableName=ScopeData2
  Scope1 : Scope
      settings: ActiveDisplayYMinimum=-1  ActiveDisplayYMaximum=1
  Sin : Trigonometry
  Sin1 : Trigonometry
  To Workspace : ToWorkspace  VariableName=ALN  SaveFormat=Timeseries  SampleTime=-1
  To Workspace1 : ToWorkspace  VariableName=ABL  SaveFormat=Timeseries  SampleTime=-1
  Transpose1 : Math  Operator=transpose
  Vector Concatenate1 : Concatenate  NumInputs=9
  Vector Concatenate3 : Concatenate  NumInputs=9
  A_BL : Outport
  wires:
  Constant3/1 -> Vector Concatenate1/8, Vector Concatenate1/7, Vector Concatenate1/6, Vector Concatenate1/3  "0"
  TA/1 -> Sin/1, Cos/1
  Gain2/1 -> Vector Concatenate1/2  "-sin(θ)"
  Sin/1 -> Vector Concatenate1/4, Gain2/1  "sin(θ)"
  Matrix Multiply/1 -> Scope/1, Transpose1/1, To Workspace/1  "A_LN"
  Cos/1 -> Vector Concatenate1/5, Vector Concatenate1/1  "cos(θ)"
  Vector Concatenate1/1 -> Reshape1/1
  Constant4/1 -> Vector Concatenate1/9  "1"
  Transpose1/1 -> Matrix Multiply2/2  "A_LN'"
  Reshape1/1 -> Matrix Multiply/1
  Reshape3/1 -> Matrix Multiply/2
  Vector Concatenate3/1 -> Reshape3/1
  Cos1/1 -> Vector Concatenate3/5, Vector Concatenate3/9  "cos(i)"
  Sin1/1 -> Vector Concatenate3/8, Gain1/1  "sin(i)"
  i/1 -> Sin1/1, Cos1/1
  Constant1/1 -> Vector Concatenate3/7, Vector Concatenate3/4, Vector Concatenate3/3, Vector Concatenate3/2  "0"
  Constant2/1 -> Vector Concatenate3/1  "1"
  Gain1/1 -> Vector Concatenate3/6  "-sin(i)"
  A_BN/1 -> Matrix Multiply2/1
  Matrix Multiply2/1 -> Scope1/1, To Workspace1/1, A_BL/1  "attitude error A_BL"
